simulink model "premikanje"  (R2021b)
settings: Solver=ode45  StartTime=0.0  StopTime=tsim  RelTol=1e-3
values from neighbouring files (symbols this model uses):
  A = [-0.0125,  0.0126,  0.0000 ... (first row only)    [main_analysis.m]    (also in main_premikanje.m; main_razstavljanje.m; main_uglasevanje.m)
  B = [-0.0091,  0.0000 ... (first row only)    [main_analysis.m]    (also in main_premikanje.m; main_razstavljanje.m; main_uglasevanje.m)
  C = [1.0, 0.0, 0.0 ... (first row only)    [main_analysis.m]    (also in main_premikanje.m; main_razstavljanje.m; main_uglasevanje.m)
  G = C*(inv(s*I-A))*B+D    [main_analysis.m]    (also in main_premikanje.m = inv(K); main_razstavljanje.m = G0*Gamma)
  integrator1_init = 0    [main_analysis.m]    (also in main_premikanje.m = 0.303; main_razstavljanje.m = 0.303; main_uglasevanje.m = 0.303)
  integrator2_init = 0    [main_analysis.m]    (also in main_premikanje.m = 0.229; main_razstavljanje.m = 0.229; main_uglasevanje.m = 0.229)
  integrator3_init = 0    [main_analysis.m]    (also in main_premikanje.m = 0.152; main_razstavljanje.m = 0.152; main_uglasevanje.m = 0.152)
  K1 = flow3_ss/(sqrt(h1_ss-h2_ss))    [main_analysis.m]    (also in main_premikanje.m; main_razstavljanje.m; main_uglasevanje.m)
  Kos1 = 9.1500    (= 9.15)    [main_analysis.m]    (also in main_premikanje.m; main_razstavljanje.m; main_uglasevanje.m)
  Kos2 = 9.6000    (= 9.6)    [main_analysis.m]    (also in main_premikanje.m; main_razstavljanje.m; main_uglasevanje.m)
  Kos3 = 9.0000    (= 9)    [main_analysis.m]    (also in main_premikanje.m; main_razstavljanje.m; main_uglasevanje.m)
  Ks1 = -27.6937    [main_analysis.m]    (also in main_premikanje.m; main_razstavljanje.m; main_uglasevanje.m)
  Ks2 = -27.5827    [main_analysis.m]    (also in main_premikanje.m; main_razstavljanje.m; main_uglasevanje.m)
  Ks3 = -27.5087    [main_analysis.m]    (also in main_premikanje.m; main_razstavljanje.m; main_uglasevanje.m)
  P = q*p    [main_premikanje.m]
  pump1_flow = [0.00000000000 0.00000000000 0.00000689390 0.00001238400 0.00001775100 0.00002311700 0.00002571800 0.00002630800 0.00002836600 0.00002892000 0.00003038100 0.00003094700 0.00003231900 0.00003196800 0.00003715200 0.00003888600 0.00004000100 0.00004024900 0.00004123900 0.00004161100 0.00004173500 0.00004179700 0.00004185800 0.00004303500 0.00004532600 0.00004644100 0.00004829800 0.00004935100 0.00005 ...(+133 chars)    [main_analysis.m]    (also in main_premikanje.m; main_razstavljanje.m; main_uglasevanje.m)
  pump1_u = [-10 -9 -8 -7 -6 -5 -4.5 -4.4 -4 -3.85 -3.6 -3.5 -3.15 -3 -2.5 -2.3 -2.1 -1.9 -1.7 -1.5 -1.3 -1.1 -0.9 -0.7 -0.5 -0.3 -0.1 0 1 2 3 4 5 6 7 8 9 10]    [main_analysis.m]    (also in main_premikanje.m; main_razstavljanje.m; main_uglasevanje.m)
  pump2_flow = [0.0000000000 0.0000000000 0.0000077952 0.0000136100 0.0000192980 0.0000248600 0.0000278520 0.0000277270 0.0000298140 0.0000305550 0.0000321400 0.0000325130 0.0000338560 0.0000350370 0.0000428520 0.0000440000 0.0000439770 0.0000448750 0.0000449380 0.0000450010 0.0000450010 0.0000450010 0.0000445510 0.0000450010 0.0000472770 0.0000496780 0.0000517010 0.0000523960 0.0000580210 0.0000630780 0.0000678 ...(+95 chars)    [main_analysis.m]    (also in main_premikanje.m; main_razstavljanje.m; main_uglasevanje.m)
  pump2_u = [-10 -9 -8 -7 -6 -5 -4.5 -4.4 -4 -3.85 -3.6 -3.5 -3.15 -3 -2.5 -2.3 -2.1 -1.9 -1.7 -1.5 -1.3 -1.1 -0.9 -0.7 -0.5 -0.3 -0.1 0 1 2 3 4 5 6 7 8 9 10]    [main_analysis.m]    (also in main_premikanje.m; main_razstavljanje.m; main_uglasevanje.m)
  r1_ss = x1_ss    (= 0.7712)    [main_premikanje.m]    (also in main_razstavljanje.m; main_uglasevanje.m)
  r2_ss = x3_ss    (= 4.8098)    [main_premikanje.m]    (also in main_razstavljanje.m; main_uglasevanje.m)
  S = 0.0152    [main_analysis.m]    (also in main_premikanje.m; main_razstavljanje.m; main_uglasevanje.m)
  u1_ss = -4    [main_analysis.m]    (also in main_premikanje.m; main_razstavljanje.m; main_uglasevanje.m)
  u2_ss = -3.5    [main_analysis.m]    (also in main_premikanje.m; main_razstavljanje.m; main_uglasevanje.m)
  u_max = 10    [main_analysis.m]    (also in main_premikanje.m; main_razstavljanje.m; main_uglasevanje.m)
  u_min = -10    [main_analysis.m]    (also in main_premikanje.m; main_razstavljanje.m; main_uglasevanje.m)
  valve3_flow = [0.0000000000 0.0000324280 0.0000360720 0.0000380760 0.0000400800 0.0000420840 0.0000429950 0.0000451810 0.0000460920 0.0000488250 0.0000499180 0.0000513750 0.0000528320 0.0000544720 0.0000562940 0.0000579610 0.0000599380 0.0000615080 0.0000630350 0.0000639460 0.0000659500 0.0000672250 0.0000695930 0.0000701400 0.0000728720 0.0000739650 0.0000748760 0.0000772450 0.0000788840 0.0000797950 0.0000828 ...(+199 chars)    [main_analysis.m]    (also in main_premikanje.m; main_razstavljanje.m; main_uglasevanje.m)
  valve3_h = [0.0000000 0.0079540 0.0146260 0.0218480 0.0294610 0.0374640 0.0457510 0.0543390 0.0632290 0.0724740 0.0820920 0.0919580 0.1021100 0.1125600 0.1233500 0.1344200 0.1458500 0.1575600 0.1695700 0.1819400 0.1945900 0.2075700 0.2208900 0.2345000 0.2484300 0.2627400 0.2772300 0.2920500 0.3072600 0.3227100 0.3385600 0.3547400 0.3711600 0.3878900 0.4050500 0.4224900 0.4400600 0.4580200 0.4762400 0.4948000 ...(+61 chars)    [main_analysis.m]    (also in main_premikanje.m; main_razstavljanje.m; main_uglasevanje.m)
  x1_ss = 0.7712    [main_analysis.m]    (also in main_premikanje.m; main_razstavljanje.m; main_uglasevanje.m)
  x2_ss = 3.2841    [main_analysis.m]    (also in main_premikanje.m; main_razstavljanje.m; main_uglasevanje.m)
  x3_ss = 4.8098    [main_analysis.m]    (also in main_premikanje.m; main_razstavljanje.m; main_uglasevanje.m)
undefined symbols (not defined in the file or in its folder): K2
libraries: spsStairGeneratorLib x2
settings Model: Creator=krist  LastModifiedBy=krist

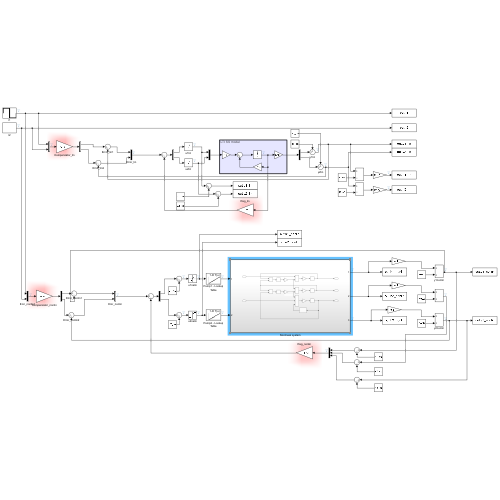
[thumbnail: Simulink's stored preview of the top-level diagram]
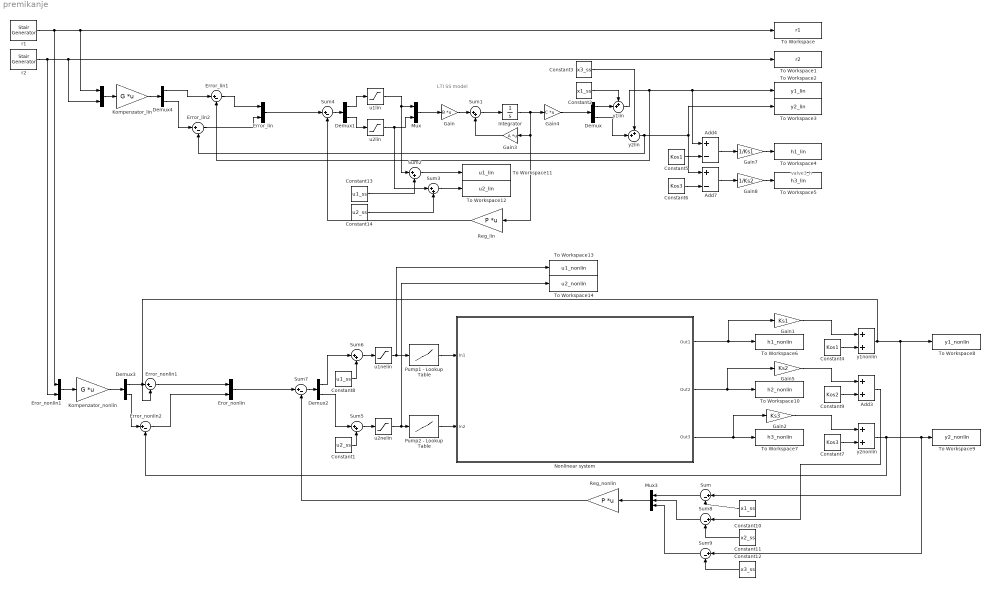
== system premikanje ==
  note: LTI SS model
  note: valve3_h
  " " : Mux  Inputs=2
  Add3 : Sum
  Add4 : Sum  Inputs=+-
  Add7 : Sum  Inputs=+-
  Constant1 : Constant  Value=u2_ss
  Constant10 : Constant  Value=x1_ss
  Constant11 : Constant  Value=x2_ss
  Constant12 : Constant  Value=x3_ss
  Constant13 : Constant  Value=u1_ss
  Constant14 : Constant  Value=u2_ss
  Constant2 : Constant  Value=x1_ss
  Constant3 : Constant  Value=x3_ss
  Constant4 : Constant  Value=Kos1
  Constant5 : Constant  Value=Kos1
  Constant6 : Constant  Value=Kos3
  Constant7 : Constant  Value=Kos3
  Constant8 : Constant  Value=u1_ss
  Constant9 : Constant  Value=Kos2
  Demux{,1..4} (5 alike) : Demux  Outputs=2
  Eror_nonlin : Mux  Inputs=2
  Eror_nonlin1 : Mux  Inputs=2
  Error_lin : Mux  Inputs=2
  Error_lin1 : Sum  Inputs=|+-
  Error_lin2 : Sum  Inputs=|+-
  Error_nonlin1 : Sum  Inputs=|+-
  Error_nonlin2 : Sum  Inputs=|+-
  Gain : Gain  Gain=B  Multiplication=Matrix(K*u)
  Gain1 : Gain  Gain=Ks1
  Gain2 : Gain  Gain=Ks3
  Gain3 : Gain  Gain=A  Multiplication=Matrix(K*u)
  Gain4 : Gain  Gain=C  Multiplication=Matrix(K*u)
  Gain5 : Gain  Gain=Ks2
  Gain7 : Gain  Gain=1/Ks1
  Gain8 : Gain  Gain=1/Ks2
  Integrator : Integrator
  Kompenzator_lin : Gain  Gain=G  Multiplication=Matrix(K*u)
  Kompenzator_nonlin : Gain  Gain=G  Multiplication=Matrix(K*u)
  Mux : Mux  Inputs=2
  Mux3 : Mux  Inputs=3
  Nonlinear system : Subsystem
  Pump1 - Lookup Table : Lookup_n-D  NumberOfTableDimensions=1  BreakpointsForDimension1=pump1_u  Table=pump1_flow  InternalRulePriority=Speed  RndMeth=Simplest  InputSameDT=on
  Pump2 - Lookup Table : Lookup_n-D  NumberOfTableDimensions=1  BreakpointsForDimension1=pump2_u  Table=pump2_flow  InternalRulePriority=Speed  RndMeth=Simplest  InputSameDT=on
  Reg_lin : Gain  Gain=P  Multiplication=Matrix(K*u)
  Reg_nonlin : Gain  Gain=P  Multiplication=Matrix(K*u)
  Sum{,4,7..9} (5 alike) : Sum  Inputs=|+-
  Sum{1..3,5..6} (5 alike) : Sum  Inputs=|++
  To Workspace : ToWorkspace  VariableName=r1  SaveFormat=Timeseries  SampleTime=-1
  To Workspace1 : ToWorkspace  VariableName=r2  SaveFormat=Timeseries  SampleTime=-1
  To Workspace10 : ToWorkspace  VariableName=h2_nonlin  SaveFormat=Timeseries  SampleTime=-1
  To Workspace11 : ToWorkspace  VariableName=u1_lin  SaveFormat=Timeseries  SampleTime=-1
  To Workspace12 : ToWorkspace  VariableName=u2_lin  SaveFormat=Timeseries  SampleTime=-1
  To Workspace13 : ToWorkspace  VariableName=u1_nonlin  SaveFormat=Timeseries  SampleTime=-1
  To Workspace14 : ToWorkspace  VariableName=u2_nonlin  SaveFormat=Timeseries  SampleTime=-1
  To Workspace2 : ToWorkspace  VariableName=y1_lin  SaveFormat=Timeseries  SampleTime=-1
  To Workspace3 : ToWorkspace  VariableName=y2_lin  SaveFormat=Timeseries  SampleTime=-1
  To Workspace4 : ToWorkspace  VariableName=h1_lin  SaveFormat=Timeseries  SampleTime=-1
  To Workspace5 : ToWorkspace  VariableName=h3_lin  SaveFormat=Timeseries  SampleTime=-1
  To Workspace6 : ToWorkspace  VariableName=h1_nonlin  SaveFormat=Timeseries  SampleTime=-1
  To Workspace7 : ToWorkspace  VariableName=h3_nonlin  SaveFormat=Timeseries  SampleTime=-1
  To Workspace8 : ToWorkspace  VariableName=y1_nonlin  SaveFormat=Timeseries  SampleTime=-1
  To Workspace9 : ToWorkspace  VariableName=y2_nonlin  SaveFormat=Timeseries  SampleTime=-1
  r1 : spsStairGeneratorLib/Stair Generator  t=r1_in.Times  e=r1_in.Vals  Ts=0
  r2 : spsStairGeneratorLib/Stair Generator  t=r2_in.Times  e=r2_in.Vals  Ts=0
  u1lin : Saturate  UpperLimit=u_max-r1_ss  LowerLimit=u_min-r1_ss
  u1nelin : Saturate  UpperLimit=u_max  LowerLimit=u_min
  u2lin : Saturate  UpperLimit=u_max-r2_ss  LowerLimit=u_min-r2_ss
  u2nelin : Saturate  UpperLimit=u_max  LowerLimit=u_min
  y1lin : Sum  Inputs=++|
  y1nonlin : Sum
  y2lin : Sum  Inputs=++|
  y2nonlin : Sum
  wires:
  r1/1 -> Eror_nonlin1/1, " "/1, To Workspace/1
  r2/1 -> Eror_nonlin1/2, " "/2, To Workspace1/1
  Demux/1 -> y1lin/2
  y1lin/1 -> Error_lin1/2, Add4/1, To Workspace2/1
  Demux/2 -> y2lin/2
  y2lin/1 -> Add7/1, To Workspace3/1, Error_lin2/2
  Constant2/1 -> y1lin/1
  Constant3/1 -> y2lin/1
  Constant5/1 -> Add4/2
  Add4/1 -> Gain7/1
  Gain7/1 -> To Workspace4/1
  Add7/1 -> Gain8/1
  Gain8/1 -> To Workspace5/1
  Constant6/1 -> Add7/2
  Pump1 - Lookup Table/1 -> Nonlinear system/1(In1)
  Pump2 - Lookup Table/1 -> Nonlinear system/2(In2)
  Nonlinear system/1(Out1) -> Gain1/1, To Workspace6/1
  Nonlinear system/3(Out3) -> Gain2/1, To Workspace7/1
  Constant7/1 -> y2nonlin/2
  Constant4/1 -> y1nonlin/2
  Gain1/1 -> y1nonlin/1
  Gain2/1 -> y2nonlin/1
  y2nonlin/1 -> Error_nonlin2/2, Sum9/1, To Workspace9/1
  y1nonlin/1 -> Sum/1, To Workspace8/1, Error_nonlin1/2
  Nonlinear system/2(Out2) -> Gain5/1, To Workspace10/1
  u1nelin/1 -> Pump1 - Lookup Table/1, To Workspace13/1
  u2nelin/1 -> To Workspace14/1, Pump2 - Lookup Table/1
  u1lin/1 -> Sum2/1, Mux/1
  u2lin/1 -> Sum3/1, Mux/2
  Sum5/1 -> u2nelin/1
  Constant1/1 -> Sum5/2
  Sum6/1 -> u1nelin/1
  Constant8/1 -> Sum6/2
  Demux1/1 -> u1lin/1
  Demux1/2 -> u2lin/1
  Error_lin1/1 -> Error_lin/1
  Error_lin2/1 -> Error_lin/2
  Demux2/1 -> Sum6/1
  Error_nonlin2/1 -> Eror_nonlin/2
  Demux2/2 -> Sum5/1
  Error_nonlin1/1 -> Eror_nonlin/1
  Mux/1 -> Gain/1
  Gain/1 -> Sum1/1
  Sum1/1 -> Integrator/1
  Gain3/1 -> Sum1/2
  Integrator/1 -> Reg_lin/1, Gain3/1, Gain4/1
  Gain4/1 -> Demux/1
  Error_lin/1 -> Sum4/1
  Sum4/1 -> Demux1/1
  Reg_lin/1 -> Sum4/2
  Gain5/1 -> Add3/1
  Constant9/1 -> Add3/2
  Eror_nonlin/1 -> Sum7/1
  Sum7/1 -> Demux2/1
  Reg_nonlin/1 -> Sum7/2
  Mux3/1 -> Reg_nonlin/1
  Sum/1 -> Mux3/1
  Sum8/1 -> Mux3/2
  Sum9/1 -> Mux3/3
  Add3/1 -> Sum8/1
  Constant10/1 -> Sum/2
  Constant11/1 -> Sum8/2
  Constant12/1 -> Sum9/2
  Sum2/1 -> To Workspace11/1
  Sum3/1 -> To Workspace12/1
  Constant13/1 -> Sum2/2
  Constant14/1 -> Sum3/2
  Eror_nonlin1/1 -> Kompenzator_nonlin/1
  Demux3/1 -> Error_nonlin1/1
  Kompenzator_nonlin/1 -> Demux3/1
  Demux3/2 -> Error_nonlin2/1
  Kompenzator_lin/1 -> Demux4/1
  " "/1 -> Kompenzator_lin/1
  Demux4/1 -> Error_lin1/1
  Demux4/2 -> Error_lin2/1

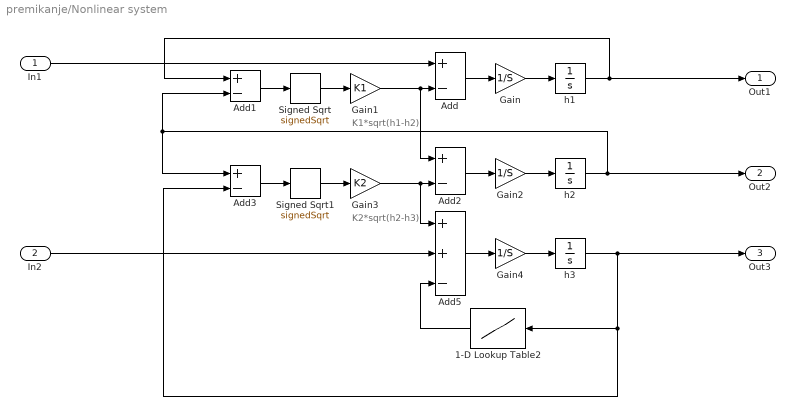
== system premikanje/Nonlinear system ==
  note: K2*sqrt(h2-h3)
  note: K1*sqrt(h1-h2)
  In1 : Inport
  In2 : Inport  Port=2
  1-D Lookup Table2 : Lookup_n-D  NumberOfTableDimensions=1  BreakpointsForDimension1=valve3_h  Table=valve3_flow  InternalRulePriority=Speed  RndMeth=Simplest  InputSameDT=on
  Add{,1..3} (4 alike) : Sum  Inputs=+-
  Add5 : Sum  Inputs=++-
  Gain : Gain  Gain=1/S
  Gain1 : Gain  Gain=K1
  Gain2 : Gain  Gain=1/S
  Gain3 : Gain  Gain=K2
  Gain4 : Gain  Gain=1/S
  Signed Sqrt : Sqrt  Operator=signedSqrt  SaturateOnIntegerOverflow=on
  Signed Sqrt1 : Sqrt  Operator=signedSqrt  SaturateOnIntegerOverflow=on
  h1 : Integrator  InitialCondition=integrator1_init
  h2 : Integrator  InitialCondition=integrator2_init
  h3 : Integrator  InitialCondition=integrator3_init
  Out1 : Outport
  Out2 : Outport  Port=2
  Out3 : Outport  Port=3
  wires:
  In2/1 -> Add5/2
  h3/1 -> Out3/1, 1-D Lookup Table2/1, Add3/2
  Add3/1 -> Signed Sqrt1/1
  Gain3/1 -> Add2/2, Add5/1
  Gain1/1 -> Add2/1, Add/2
  Add2/1 -> Gain2/1
  Gain4/1 -> h3/1
  Gain2/1 -> h2/1
  h2/1 -> Out2/1, Add1/2, Add3/1
  Add1/1 -> Signed Sqrt/1
  Add/1 -> Gain/1
  h1/1 -> Out1/1, Add1/1
  Gain/1 -> h1/1
  Add5/1 -> Gain4/1
  In1/1 -> Add/1
  Signed Sqrt/1 -> Gain1/1
  1-D Lookup Table2/1 -> Add5/3
  Signed Sqrt1/1 -> Gain3/1
